simulink model "ppi_ctrl2"  (R2020b)
settings: Solver=VariableStepAuto  StartTime=0.0  StopTime=10.0  RelTol=1e-3
values from neighbouring files (symbols this model uses):
  a1 = 1    [script_ppi.m]
  g = [g1;g2]    [robo.m]    (also in script_ppi.m = 9.8)
  Il = [Il1 Il2]    [script_ppi.m]
  Im = [Im1 Im2]    [script_ppi.m]
  Ka = M_    [ppi_tuning.m]
  Kd = deltad1(2)*M_    [ppi_tuning.m]
  Ki = deltad1(3)*M_    [ppi_tuning.m]
  Kp = deltad2(1)/deltad1(3)    [ppi_tuning.m]    (also in script_ppi.m = double(Kp))
  Kr = [Kr1 Kr2]    [script_ppi.m]
  l = [l1 l2]    [script_ppi.m]
  l2 = 0.5    [robo.m]    (also in script_ppi.m)
  ml = [ml1 ml2]    [script_ppi.m]
  ml2 = 60    [script_ppi.m]
  mm = [mm1 mm2]    [script_ppi.m]
  q0 = [0 0 0 0]'    [script_ppi.m]
undefined symbols (not defined in the file or in its folder): traj_switch
settings Model: Creator=lucas  LastModifiedBy=lucas

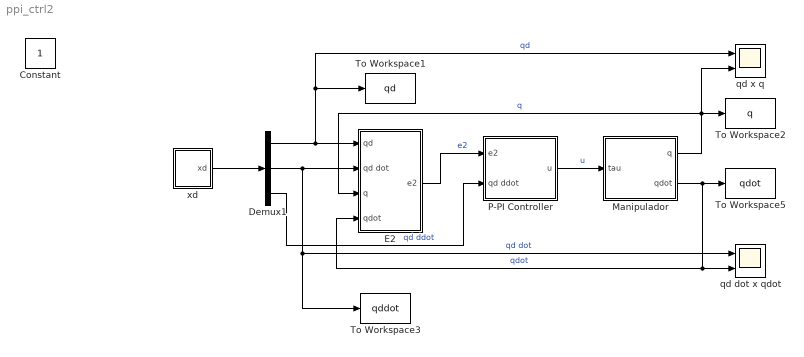
== system ppi_ctrl2 ==
  Demux1 : Demux  Outputs=3
  E2 : Subsystem
  Manipulador : Subsystem
  P-PI Controller : Subsystem
  To Workspace1 : ToWorkspace  VariableName=qd  SaveFormat=Timeseries  SampleTime=-1
  To Workspace2 : ToWorkspace  VariableName=q  SaveFormat=Timeseries  SampleTime=-1
  To Workspace3 : ToWorkspace  VariableName=qddot  SaveFormat=Timeseries  SampleTime=-1
  To Workspace5 : ToWorkspace  VariableName=qdot  SaveFormat=Timeseries  SampleTime=-1
  qd dot x qdot : Scope  NumInputPorts=2
  qd x q : Scope  NumInputPorts=2
  xd : Subsystem
  Constant : Constant  IOType=siggen
  wires:
  Manipulador/1(q) -> To Workspace2/1, qd x q/2, E2/3(q)  "q"
  Demux1/1 -> qd x q/1, To Workspace1/1, E2/1(qd)  "qd"
  Demux1/2 -> qd dot x qdot/1, To Workspace3/1, E2/2(qd dot)  "qd dot"
  Manipulador/2(qdot) -> To Workspace5/1, qd dot x qdot/2, E2/4(qdot)  "qdot"
  E2/1(e2) -> P-PI Controller/1(e2)  "e2"
  Demux1/3 -> P-PI Controller/2(qd ddot)  "qd ddot"
  P-PI Controller/1(u) -> Manipulador/1(tau)  "u"
  xd/1(xd) -> Demux1/1

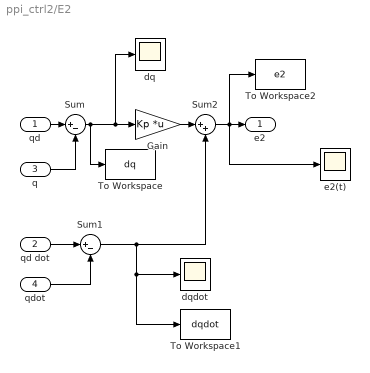
== system ppi_ctrl2/E2 ==
  qd : Inport
  qd dot : Inport  Port=2
  q : Inport  Port=3
  qdot : Inport  Port=4
  Gain : Gain  Gain=Kp  Multiplication=Matrix(K*u)
  Sum : Sum  Inputs=|+-
  Sum1 : Sum  Inputs=|+-
  Sum2 : Sum  Inputs=|++
  To Workspace : ToWorkspace  VariableName=dq  SaveFormat=Timeseries  SampleTime=-1
  To Workspace1 : ToWorkspace  VariableName=dqdot  SaveFormat=Timeseries  SampleTime=-1
  To Workspace2 : ToWorkspace  VariableName=e2  SaveFormat=Timeseries  SampleTime=-1
  dq : Scope
  dqdot : Scope
  e2(t) : Scope
  e2 : Outport
  wires:
  Sum/1 -> To Workspace/1, dq/1, Gain/1
  Sum1/1 -> To Workspace1/1, dqdot/1, Sum2/2
  qdot/1 -> Sum1/2
  q/1 -> Sum/2
  Gain/1 -> Sum2/1
  qd/1 -> Sum/1
  qd dot/1 -> Sum1/1
  Sum2/1 -> e2(t)/1, To Workspace2/1, e2/1

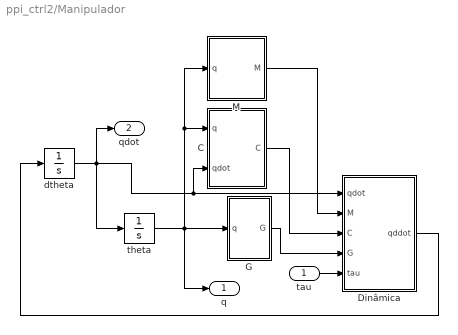
== system ppi_ctrl2/Manipulador ==
  tau : Inport
  C : Subsystem
  Dinâmica : MATLAB Function  TreatAsAtomicUnit=on
  G : Subsystem
  M : Subsystem
  dtheta : Integrator  InitialCondition=q0(3:4)
  theta : Integrator  InitialCondition=q0(1:2)
  q : Outport
  qdot : Outport  Port=2
  wires:
  C/1(C) -> Dinâmica/3(C)
  dtheta/1 -> qdot/1, C/2(qdot), Dinâmica/1(qdot), theta/1
  theta/1 -> q/1, M/1(q), C/1(q), G/1(q)
  M/1(M) -> Dinâmica/2(M)
  tau/1 -> Dinâmica/5(tau)
  Dinâmica/1(qddot) -> dtheta/1
  G/1(G) -> Dinâmica/4(G)

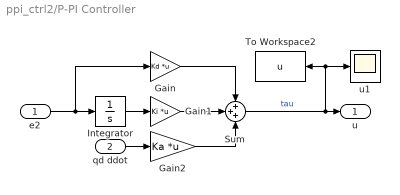
== system ppi_ctrl2/P-PI Controller ==
  e2 : Inport
  qd ddot : Inport  Port=2
  Gain : Gain  Gain=Kd  Multiplication=Matrix(K*u)
  Gain1 : Gain  Gain=Ki  Multiplication=Matrix(K*u)
  Gain2 : Gain  Gain=Ka  Multiplication=Matrix(K*u)
  Integrator : Integrator
  Sum : Sum  Inputs=+++
  To Workspace2 : ToWorkspace  VariableName=u  SaveFormat=Timeseries  SampleTime=-1
  u1 : Scope
  u : Outport
  wires:
  Gain1/1 -> Sum/2
  qd ddot/1 -> Gain2/1
  Gain2/1 -> Sum/3
  Gain/1 -> Sum/1
  Integrator/1 -> Gain1/1
  e2/1 -> Gain/1, Integrator/1
  Sum/1 -> u1/1, To Workspace2/1, u/1  "tau"

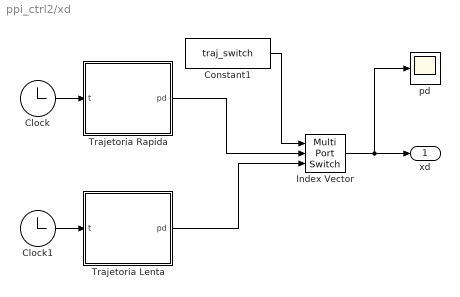
== system ppi_ctrl2/xd ==
  Clock : Clock
  Clock1 : Clock
  Constant1 : Constant  Value=traj_switch
  Index Vector : MultiPortSwitch  DataPortOrder=Zero-based contiguous  Inputs=2  zeroidx=on
  Trajetoria Lenta : MATLAB Function  TreatAsAtomicUnit=on
  Trajetoria Rapida : MATLAB Function  TreatAsAtomicUnit=on
  pd : Scope
  xd : Outport
  wires:
  Trajetoria Lenta/1(pd) -> Index Vector/3
  Clock/1 -> Trajetoria Rapida/1(t)
  Constant1/1 -> Index Vector/1
  Trajetoria Rapida/1(pd) -> Index Vector/2
  Clock1/1 -> Trajetoria Lenta/1(t)
  Index Vector/1 -> pd/1, xd/1

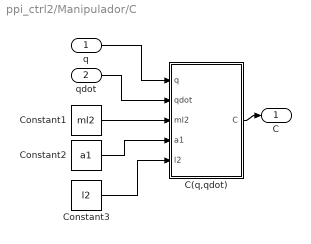
== system ppi_ctrl2/Manipulador/C ==
  q : Inport
  qdot : Inport  Port=2
  C(q,qdot) : MATLAB Function  TreatAsAtomicUnit=on
  Constant1 : Constant  Value=ml2
  Constant2 : Constant  Value=a1
  Constant3 : Constant  Value=l2
  C : Outport
  wires:
  C(q,qdot)/1(C) -> C/1
  Constant2/1 -> C(q,qdot)/4(a1)
  Constant3/1 -> C(q,qdot)/5(l2)
  Constant1/1 -> C(q,qdot)/3(ml2)
  q/1 -> C(q,qdot)/1(q)
  qdot/1 -> C(q,qdot)/2(qdot)

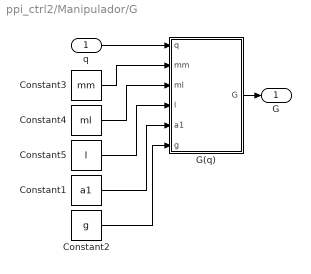
== system ppi_ctrl2/Manipulador/G ==
  q : Inport
  Constant1 : Constant  Value=a1
  Constant2 : Constant  Value=g
  Constant3 : Constant  Value=mm
  Constant4 : Constant  Value=ml
  Constant5 : Constant  Value=l
  G(q) : MATLAB Function  TreatAsAtomicUnit=on
  G : Outport
  wires:
  Constant4/1 -> G(q)/3(ml)
  G(q)/1(G) -> G/1
  Constant3/1 -> G(q)/2(mm)
  Constant5/1 -> G(q)/4(l)
  q/1 -> G(q)/1(q)
  Constant1/1 -> G(q)/5(a1)
  Constant2/1 -> G(q)/6(g)

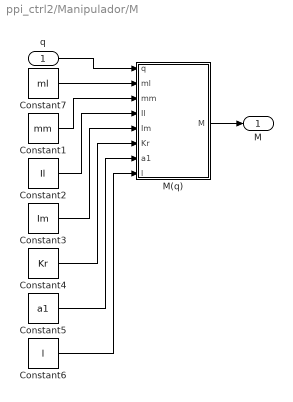
== system ppi_ctrl2/Manipulador/M ==
  q : Inport
  Constant1 : Constant  Value=mm
  Constant2 : Constant  Value=Il
  Constant3 : Constant  Value=Im
  Constant4 : Constant  Value=Kr
  Constant5 : Constant  Value=a1
  Constant6 : Constant  Value=l
  Constant7 : Constant  Value=ml
  M(q) : MATLAB Function  TreatAsAtomicUnit=on
  M : Outport
  wires:
  Constant3/1 -> M(q)/5(Im)
  Constant2/1 -> M(q)/4(Il)
  Constant1/1 -> M(q)/3(mm)
  M(q)/1(M) -> M/1
  Constant4/1 -> M(q)/6(Kr)
  Constant5/1 -> M(q)/7(a1)
  q/1 -> M(q)/1(q)
  Constant6/1 -> M(q)/8(l)
  Constant7/1 -> M(q)/2(ml)

== matlab function ppi_ctrl2/Manipulador/C/C(q,qdot) ==
  data: q input; qdot input; C output; ml2 input; a1 input; l2 input
function C = fcn(q,qdot,ml2,a1,l2)
    h = -ml2*a1*l2*sin(q(2));
    c11 = h*qdot(2);
    c12 = h*(qdot(1) + qdot(2));
    c21 = -h*qdot(1);
    c22 = 0;
    C = [c11 c12;
        c21 c22
        ];
end

== matlab function ppi_ctrl2/Manipulador/M/M(q) ==
  data: q input; ml input; M output; mm input; Il input; Im input; Kr input; a1 input; l input
function M = fcn(q,ml,mm,Il,Im,Kr,a1,l)
    q1 = q(1);
    q2 = q(2);
    
    mm1 = mm(1);
    mm2 = mm(2);
    
    ml1 = ml(1);
    ml2 = ml(2);
    
    Im1 = Im(1);
    Im2 = Im(2);
    
    Il1 = Il(1);
    Il2 = Il(2);
    
    l1 = l(1);
    l2 = l(2);
    
    Kr1 = Kr(1);
    Kr2 = Kr(2);
    
    % M matrix
    b11 = Il1+ml1*l1^2+(Kr1^2)*Im1+Il2+ml2*(a1^2+l2^2+2*a1*l2*cos(q(2)))+Im2+mm2*a1^2;
    b12 = Il2 + ml2*(l2^2 +a1*l2*cos(q(2))) + Kr2*Im2;
    b22 = Il2 + ml2^2 + Kr2^2*Im2;

    M = [
        b11 b12;
        b12 b22
        ];
end

== matlab function ppi_ctrl2/Manipulador/G/G(q) ==
  data: q input; G output; mm input; ml input; l input; a1 input; g input
function G = fcn(q,mm,ml,l,a1,g)
    ml1 = ml(1);
    ml2 = ml(2);
    
    mm1 = mm(1);
    mm2 = mm(2);
    
    l1 = l(1);
    l2 = l(2);
    
    G1 = mm1*l1 + mm2*a1 + ml2*a1*g*cos(q(1)) + ml2*l2*g*cos(q(1)+q(2));
    G2 = ml2*l2*g*cos(q(1) + q(2));
    
    G = [G1;
         G2
        ];
end

== matlab function ppi_ctrl2/Manipulador/Dinâmica ==
  data: qddot output; qdot input; M input; C input; G input; tau input
function qddot = fcn(qdot,M,C,G,tau)
    qddot = -inv(M)*(C*qdot+G-tau);
end

== matlab function ppi_ctrl2/xd/Trajetoria Lenta ==
  data: pd output; t input
function pd = fcn(t)
qd = [(-0.75*cos(pi*t/2))-0.75; (-0.75*cos(pi*t/2))+3.75];

qddot = [0.75*(pi/2)*sin(pi*t/2); 0.75*(pi/2)*sin(pi*t/2)];

qdddot = [0.75*(pi/2)^2*cos(pi*t/2); 0.75*(pi/2)^2*cos(pi*t/2)];

pd = [qd;qddot;qdddot];

== matlab function ppi_ctrl2/xd/Trajetoria Rapida ==
  data: pd output; t input
function pd = fcn(t)
qd = [(-0.75*cos(pi*t))-0.75; (-0.75*cos(pi*t))+3.75];

qddot = [0.75*pi*sin(pi*t); 0.75*pi*sin(pi*t)];

qdddot = [0.75*pi^2*cos(pi*t); 0.75*pi^2*cos(pi*t)];

pd = [qd;qddot;qdddot];
